simulink library "Spring_Control_Hydropneumatic"  (R2023a)
settings: Solver=VariableStepAuto  StartTime=0.0  StopTime=10.0  RelTol=1e-3
libraries: Vehicle_Outputs x1
Description:
  | Copyright 2026 The MathWorks, Inc.
settings Model: Creator=smiller  LastModifiedBy=smiller
settings OptimizationCC: ReuseModelBlockBuffer=off
settings ModelReferenceCC: EnableRefExpFcnMdlSchedulingChecks=on

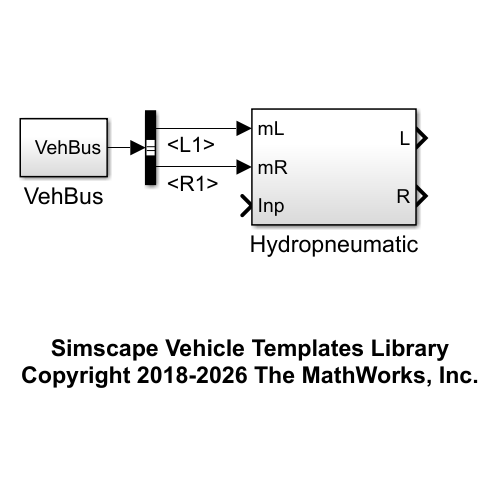
[thumbnail: Simulink's stored preview of the top-level diagram]
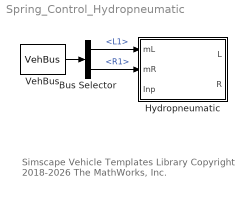
== system Spring_Control_Hydropneumatic ==
  note: Simscape Vehicle Templates Library
      | Copyright 2018-2026 The MathWorks, Inc.
  Bus Selector : BusSelector  OutputSignals=Chassis.Damper.L1,Chassis.Damper.R1
  Hydropneumatic : Subsystem  VariantControl=Choice
  VehBus : Vehicle_Outputs/VehBus  SystemSampleTime=-1  VariantActivationTime=update diagram  Latency=0  AutoFrameSizeCalculation=off
  wires:
  VehBus/1 -> Bus Selector/1
  Bus Selector/1 -> Hydropneumatic/1(mL)  "<L1>"
  Bus Selector/2 -> Hydropneumatic/2(mR)  "<R1>"

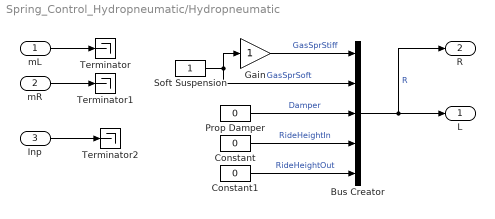
== system Spring_Control_Hydropneumatic/Hydropneumatic ==
  mL : Inport
  mR : Inport  Port=2
  Inp : Inport  Port=3
  Bus Creator : BusCreator  Inputs=5
  Constant : Constant  Value=0
  Constant1 : Constant  Value=0
  Gain : Gain
  Prop Damper : Constant  Value=0
  Soft Suspension : Constant
  Terminator : Terminator
  Terminator1 : Terminator
  Terminator2 : Terminator
  L : Outport  VectorParamsAs1DForOutWhenUnconnected=off
  R : Outport  Port=2  VectorParamsAs1DForOutWhenUnconnected=off
  wires:
  Bus Creator/1 -> R/1, L/1  "R"
  mL/1 -> Terminator/1
  mR/1 -> Terminator1/1
  Inp/1 -> Terminator2/1
  Constant1/1 -> Bus Creator/5  "RideHeightOut"
  Gain/1 -> Bus Creator/1  "GasSprStiff"
  Soft Suspension/1 -> Bus Creator/2, Gain/1  "GasSprSoft"
  Prop Damper/1 -> Bus Creator/3  "Damper"
  Constant/1 -> Bus Creator/4  "RideHeightIn"
